simulink model "untitled"  (Simulink 6.4)
settings: Solver=ode45  StartTime=0.0  StopTime=inf  RelTol=1e-3
libraries: simulink x3
settings Model: LastModifiedBy=Maggia

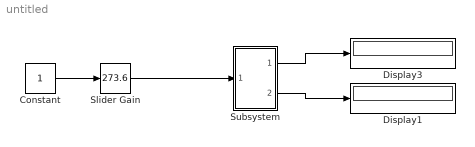
== system untitled ==
  Constant : Constant  Value=1  OutDataType=sfix(16)  ConRadixGroup=Use specified scaling  OutScaling=2^0  SampleTime=inf  FramePeriod=inf
  Display1 : Display
  Display3 : Display
  Slider Gain : simulink/Math Operations/Slider Gain  SystemSampleTime=-1  low=0  gain=273.6  high=360
  Subsystem : Subsystem
  wires:
  Constant/1 -> Slider Gain/1
  Slider Gain/1 -> Subsystem/1(In1)
  Subsystem/1(Out1) -> Display3/1
  Subsystem/2(Out2) -> Display1/1

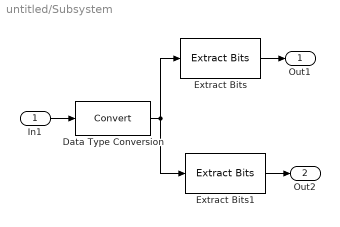
== system untitled/Subsystem ==
  In1 : Inport
  Data Type Conversion : DataTypeConversion  OutDataTypeMode=uint16
  Extract Bits : simulink/Logic and Bit Operations/Extract Bits  SystemSampleTime=-1  bitsToExtract=Range of bits  numBits=8  bitIdxRange=[0 7]  outScalingMode=Treat bit field as an integer
  Extract Bits1 : simulink/Logic and Bit Operations/Extract Bits  SystemSampleTime=-1  bitsToExtract=Range of bits  numBits=8  bitIdxRange=[8 15]  outScalingMode=Treat bit field as an integer
  Out1 : Outport
  Out2 : Outport  Port=2
  wires:
  Data Type Conversion/1 -> Extract Bits1/1, Extract Bits/1
  Extract Bits/1 -> Out1/1
  In1/1 -> Data Type Conversion/1
  Extract Bits1/1 -> Out2/1
